simulink model "sim_validation_6DoF_3DoF"  (R2025a)
settings: Solver=VariableStepAuto  StartTime=0.0  StopTime=tf  RelTol=1e-12  AbsTol=1e-12
values from neighbouring files (symbols this model uses):
  alpha = 0.5086    [3DoF_deterministic_Workspace.mat]    (also in Compressed_Time_Step_2dof_Experiment.mat; Copy_of_Deterministic_6DoF.m; Copy_of_Deterministic_6DoF_quat.m; Copy_of_SCP_Earth_Mars_transfer_GA_uniform_adaptive.m = 1)
  I = 0.15    [3DoF_deterministic_Workspace.mat]    (also in Copy_of_DQG_6DoF_fixedtf.m = [4.2; 4.2; 0.6]; Copy_of_Deterministic_6DoF.m = [50000; 150000; 150000] * (1e-3) ^ 2; Copy_of_Deterministic_6DoF_quat.m = [50000; 150000; 150000] * (1e-3) ^ 2; DQG_6DoF.m = [4.2; 4.2; 0.6])
  I_matrix = diag([I/5, I, I])    [Deterministic_3DoF_with_mass_convexified_reynolds.m]    (also in Deterministic_3DoF_with_mass_convexified_takeoffdivert.m; Deterministic_6DoF.m = diag(I); Deterministic_6DoF_reynolds.m = diag(I); Deterministic_6DoF_reynolds_quat_alphabeta.m = diag(I))
  input_vector = 1:nu    [Deterministic_3DoF_with_mass_convexified_reynolds.m]    (also in Deterministic_3DoF_with_mass_convexified_takeoffdivert.m; Deterministic_3DoF_with_mass_polar.m; Deterministic_6DoF.m; Deterministic_6DoF_reynolds.m)
  L = 0.003    [3DoF_deterministic_Workspace.mat]    (also in Compressed_Time_Step_2dof_Experiment.mat; Copy_of_DQG_6DoF_fixedtf.m = 1; Copy_of_Deterministic_6DoF.m; Copy_of_Deterministic_6DoF_quat.m)
  m_0 = 2100    [3DoF_deterministic_Workspace.mat]    (also in Compressed_Time_Step_2dof_Experiment.mat = 2000; Copy_of_Deterministic_6DoF.m = 2600; Copy_of_Deterministic_6DoF_quat.m = 2600; Copy_of_SCP_Earth_Mars_transfer_GA_uniform_adaptive.m = 1)
  m_dry = 1500    [3DoF_deterministic_Workspace.mat]    (also in Copy_of_Deterministic_6DoF.m = 2000; Copy_of_Deterministic_6DoF_quat.m = 2000; Deterministic_3DoF.m = 2000; Deterministic_3DoF_with_mass.m)
  m_wet = 600    [3DoF_deterministic_Workspace.mat]    (also in Copy_of_Deterministic_6DoF.m; Copy_of_Deterministic_6DoF_quat.m; Deterministic_3DoF.m; Deterministic_3DoF_with_mass.m)
  r_0_6DoF = [r_0(1); 0; r_0(2)]    [Deterministic_3DoF_with_mass_convexified_reynolds.m]    (also in Deterministic_3DoF_with_mass_convexified_takeoffdivert.m; Deterministic_6DoF.m = r_0; Deterministic_6DoF_reynolds.m = r_0; Deterministic_6DoF_reynolds_quat_alphabeta.m = r_0)
  rpy_0_6DoF = [0; theta_0; 0]    [Deterministic_3DoF_with_mass_convexified_reynolds.m]    (also in Deterministic_3DoF_with_mass_convexified_takeoffdivert.m; Deterministic_6DoF.m = dcm2angle(angle2dcm(theta1_0, theta2_0, theta3_0,"XYX"), "ZY; Deterministic_6DoF_reynolds.m = dcm2angle(angle2dcm(theta1_0, theta2_0, theta3_0,"XYX"), "ZY; Deterministic_6DoF_reynolds_quat_alphabeta.m = [theta_3; theta_1; theta_2])
  v_0_b_6DoF = [v_0_b(1); 0; v_0_b(2)]    [Deterministic_3DoF_with_mass_convexified_reynolds.m]    (also in Deterministic_3DoF_with_mass_convexified_takeoffdivert.m; Deterministic_6DoF.m = v_0_b; Deterministic_6DoF_reynolds.m = v_0_b; Deterministic_6DoF_reynolds_quat_alphabeta.m = quat_rot(q_conj(q_0), v_0))
  w_0_6DoF = [0; w_0; 0]    [Deterministic_3DoF_with_mass_convexified_reynolds.m]    (also in Deterministic_3DoF_with_mass_convexified_takeoffdivert.m; Deterministic_6DoF.m = w_0; Deterministic_6DoF_reynolds.m = w_0; Deterministic_6DoF_reynolds_quat_alphabeta.m = w_0)
  x_0_6DoF = [r_0_6DoF; v_0_6DoF; rpy_0_6DoF; w_0_6DoF; log(m_0)]    [Deterministic_3DoF_with_mass_convexified_reynolds.m]    (also in Deterministic_3DoF_with_mass_convexified_takeoffdivert.m; Deterministic_6DoF.m = [r_0_6DoF; v_0_6DoF; rpy_0_6DoF; w_0_6DoF]; Deterministic_6DoF_reynolds.m = [r_0_6DoF; v_0_6DoF; rpy_0_6DoF; w_0_6DoF]; Deterministic_6DoF_reynolds_quat_alphabeta.m = x_0)
undefined symbols (not defined in the file or in its folder): construct_dual_quat
libraries: sharedtransform x2, simulink_extras x2, aerolibanim x1, aerolibobsolete x1, aerolibanimutils x1
settings Model: Creator=thatf  LastModifiedBy=thatf

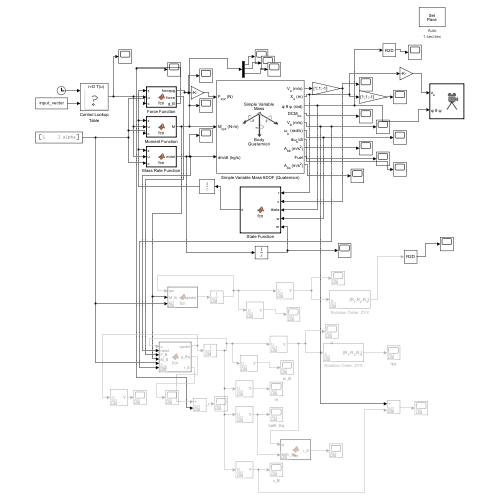
[thumbnail: Simulink's stored preview of the top-level diagram]
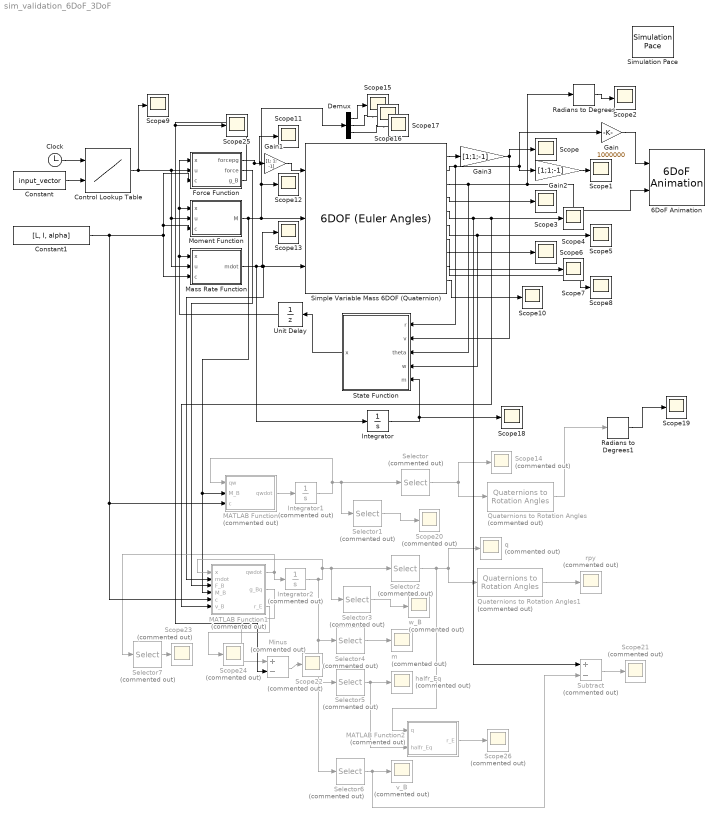
== system sim_validation_6DoF_3DoF ==
  6DoF Animation : aerolibanim/6DoF Animation  u1=[-1000 1000 -1000 1000 -5000 50]  u2=0.05  u3=100  u4=[0 0 0]  u5=Fly alongside  u6=[0 1000 0]  u7=80  u8=on
  Clock : Clock
  Constant : Constant  Value=input_vector
  Constant1 : Constant  Value=[L, I, alpha]
  Control Lookup Table : Lookup_n-D  BreakpointsForDimension1=opt_time'  BreakpointsForDimension2=input_vector  Table=control_inputs'  InternalRulePriority=Speed  RndMeth=Simplest
      settings: InputPortMap=u0,u1
  Demux : Demux  Outputs=3
  Force Function : MATLAB Function  TreatAsAtomicUnit=on
  Gain : Gain  Gain=1000000
  Gain1 : Gain  Gain=[1; 1; -1]
  Gain2 : Gain  Gain=[1;1;-1]
  Gain3 : Gain  Gain=[1;1;-1]
  Integrator : Integrator  InitialCondition=m_0
  Integrator1 : Integrator  Commented=on  InitialCondition=[[0 1 0 0; 0 0 1 0; 0 0 0 1; 1 0 0 0] * angle2quat(rpy_0_6DoF(1), rpy_0_6DoF(2), rpy_0_6DoF(3))'; w_0_6DoF]
  Integrator2 : Integrator  Commented=on  InitialCondition=[m_0; construct_dual_quat([0 1 0 0; 0 0 1 0; 0 0 0 1; 1 0 0 0] * angle2quat(rpy_0_6DoF(1), rpy_0_6DoF(2), rpy_0_6DoF(3))', r_0_6DoF); w_0_6DoF; v_0_b_6DoF]
  MATLAB Function : MATLAB Function  Commented=on  TreatAsAtomicUnit=on
  MATLAB Function1 : MATLAB Function  Commented=on  TreatAsAtomicUnit=on
  MATLAB Function2 : MATLAB Function  Commented=on  TreatAsAtomicUnit=on
  Mass Rate Function : MATLAB Function  TreatAsAtomicUnit=on
  Minus : Sum  Commented=on  Inputs=+-
  Moment Function : MATLAB Function  TreatAsAtomicUnit=on
  Quaternions to Rotation Angles : sharedtransform/Quaternions to Rotation Angles  Commented=on  rotationOrder=ZYX  aMode=aMode
  Quaternions to Rotation Angles1 : sharedtransform/Quaternions to Rotation Angles  Commented=on  rotationOrder=ZYX  aMode=aMode
  Radians to Degrees : simulink_extras/Transformations/Radians to Degrees
  Radians to Degrees1 : simulink_extras/Transformations/Radians to Degrees
  Scope{,1..13,15..19,25} (20 alike) : Scope
      Scope settings: ActiveDisplayYMinimum=-0.67191  ActiveDisplayYMaximum=-0.0103
      Scope1 settings: ActiveDisplayYMinimum=-7.33016  ActiveDisplayYMaximum=5.92557
      Scope10 settings: ActiveDisplayYMinimum=-0.01134  ActiveDisplayYMaximum=0.0087  DataLoggingVariableName=ScopeData2
      Scope11 settings: ActiveDisplayYMinimum=-25.88331  ActiveDisplayYMaximum=91.30016
      Scope12 settings: ActiveDisplayYMinimum=-0.01345  ActiveDisplayYMaximum=0.01341  DataLoggingVariableName=ScopeData2
      Scope13 settings: ActiveDisplayYMinimum=-33.22212  ActiveDisplayYMaximum=-15.43213  DataLoggingVariableName=ScopeData3
      Scope15 settings: ActiveDisplayYMinimum=-1  ActiveDisplayYMaximum=1  DataLoggingVariableName=ScopeData2
      Scope16 settings: ActiveDisplayYMinimum=-0.01345  ActiveDisplayYMaximum=0.01341  DataLoggingVariableName=ScopeData3
      Scope17 settings: ActiveDisplayYMinimum=-1  ActiveDisplayYMaximum=1  DataLoggingVariableName=ScopeData4
      Scope18 settings: ActiveDisplayYMinimum=1344.12679  ActiveDisplayYMaximum=2183.98591  DataLoggingVariableName=ScopeData5
      Scope19 settings: ActiveDisplayYMinimum=-1  ActiveDisplayYMaximum=1  DataLoggingVariableName=ScopeData2
      Scope2 settings: ActiveDisplayYMinimum=-225  ActiveDisplayYMaximum=225  DataLoggingVariableName=ScopeData2
      Scope25 settings: ActiveDisplayYMinimum=-0.01099  ActiveDisplayYMaximum=0.01074  DataLoggingVariableName=ScopeData15
      Scope3 settings: ActiveDisplayYMinimum=-1.25  ActiveDisplayYMaximum=1.25  DataLoggingVariableName=ScopeData3
      Scope4 settings: ActiveDisplayYMinimum=-0.68624  ActiveDisplayYMaximum=0.36359  DataLoggingVariableName=ScopeData4
      Scope5 settings: ActiveDisplayYMinimum=-0.26753  ActiveDisplayYMaximum=0.38262  DataLoggingVariableName=ScopeData5
      Scope6 settings: ActiveDisplayYMinimum=-0.08967  ActiveDisplayYMaximum=0.08939  DataLoggingVariableName=ScopeData6
      Scope7 settings: ActiveDisplayYMinimum=-0.18108  ActiveDisplayYMaximum=0.11428  DataLoggingVariableName=ScopeData7
      Scope8 settings: ActiveDisplayYMinimum=-0.125  ActiveDisplayYMaximum=1.125  DataLoggingVariableName=ScopeData8
      Scope9 settings: ActiveDisplayYMinimum=-0.00667  ActiveDisplayYMaximum=0.03493
  Scope{14,20..24,26} (7 alike) : Scope  Commented=on
      Scope14 settings: ActiveDisplayYMinimum=-0.12098  ActiveDisplayYMaximum=1.08883
      Scope20 settings: ActiveDisplayYMinimum=-0.38229  ActiveDisplayYMaximum=0.26726  DataLoggingVariableName=ScopeData3
      Scope21 settings: ActiveDisplayYMinimum=-0.04069  ActiveDisplayYMaximum=0.03672  DataLoggingVariableName=ScopeData11
      Scope22 settings: ActiveDisplayYMinimum=-6E-5  ActiveDisplayYMaximum=9E-5  DataLoggingVariableName=ScopeData12
      Scope23 settings: ActiveDisplayYMinimum=-0.03752  ActiveDisplayYMaximum=0.04457  DataLoggingVariableName=ScopeData13
      Scope24 settings: ActiveDisplayYMinimum=-0.64016  ActiveDisplayYMaximum=5.18224  DataLoggingVariableName=ScopeData14
      Scope26 settings: ActiveDisplayYMinimum=-5.29494  ActiveDisplayYMaximum=1.65449  DataLoggingVariableName=ScopeData9
  Selector : Selector  Commented=on  InputPortWidth=7  IndexOptions=Index vector (dialog)  Indices=[4 1 2 3]  OutputSizes=1
  Selector1 : Selector  Commented=on  InputPortWidth=7  IndexOptions=Index vector (dialog)  Indices=[5:7]  OutputSizes=1
  Selector2 : Selector  Commented=on  InputPortWidth=15  IndexOptions=Index vector (dialog)  Indices=[5 2 3 4]  OutputSizes=1
  Selector3 : Selector  Commented=on  InputPortWidth=15  IndexOptions=Index vector (dialog)  Indices=[10:12]  OutputSizes=1
  Selector4 : Selector  Commented=on  InputPortWidth=15  IndexOptions=Index vector (dialog)  Indices=[1]  OutputSizes=1
  Selector5 : Selector  Commented=on  InputPortWidth=15  IndexOptions=Index vector (dialog)  Indices=[6:9]  OutputSizes=1
  Selector6 : Selector  Commented=on  InputPortWidth=15  IndexOptions=Index vector (dialog)  Indices=[13:15]  OutputSizes=1
  Selector7 : Selector  Commented=on  InputPortWidth=15  IndexOptions=Index vector (dialog)  Indices=[13:15]  OutputSizes=1
  Simple Variable Mass 6DOF (Quaternion) : aerolibobsolete/6DOF (Euler Angles)  units=Metric (MKS)  mtype=Simple Variable  rep=Quaternion  xme_0=r_0_6DoF .* [1; 1; -1]  Vm_0=v_0_b_6DoF .* [1; 1; -1]  eul_0=rpy_0_6DoF  pm_0=w_0_6DoF  mass_0=m_0  mass_e=m_dry  mass_f=m_wet + m_dry  inertia=eye(3)  inertia_e=I_matrix - 1e-12  inertia_f=I_matrix  k_quat=1.0  vre_flag=off  abi_flag=on  aMode=0  xme_statename=''  Vm_statename=''  eul_statename=''  quat_statename=''  pm_statename=''  mass_statename=''
  Simulation Pace : aerolibanimutils/Simulation Pace  SimulationPace=1  SleepMode=Auto  OutputPaceError=off  SampleTime=1/30
  State Function : MATLAB Function  TreatAsAtomicUnit=on
  Subtract : Sum  Commented=on  Inputs=+-
  Unit Delay : UnitDelay  InitialCondition=x_0_6DoF  SampleTime=-1  HasFrameUpgradeWarning=on
  halfr_Eq : Scope  Commented=on
      settings: ActiveDisplayYMinimum=-2.39  ActiveDisplayYMaximum=1.59146  DataLoggingVariableName=ScopeData8
  m : Scope  Commented=on
      settings: ActiveDisplayYMinimum=1344.12679  ActiveDisplayYMaximum=2183.98591  DataLoggingVariableName=ScopeData7
  q : Scope  Commented=on
      settings: ActiveDisplayYMinimum=-0.12098  ActiveDisplayYMaximum=1.08883  DataLoggingVariableName=ScopeData4
  rpy : Scope  Commented=on
      settings: ActiveDisplayYMinimum=-0.3927  ActiveDisplayYMaximum=3.53429  DataLoggingVariableName=ScopeData6
  v_B : Scope  Commented=on
      settings: ActiveDisplayYMinimum=-0.34837  ActiveDisplayYMaximum=0.07536  DataLoggingVariableName=ScopeData10
  w_B : Scope  Commented=on
      settings: ActiveDisplayYMinimum=-0.38229  ActiveDisplayYMaximum=0.26726  DataLoggingVariableName=ScopeData5
  wires:
  Mass Rate Function/1(mdot) -> MATLAB Function1/2(mdot), Simple Variable Mass 6DOF (Quaternion)/3, Scope13/1, Integrator/1
  Simple Variable Mass 6DOF (Quaternion)/3 -> State Function/3(theta), 6DoF Animation/2, Radians to Degrees/1
  Simple Variable Mass 6DOF (Quaternion)/4 -> Scope3/1
  Simple Variable Mass 6DOF (Quaternion)/6 -> State Function/4(w), Scope5/1
  Simple Variable Mass 6DOF (Quaternion)/7 -> Scope6/1
  Simple Variable Mass 6DOF (Quaternion)/8 -> Scope7/1
  Simple Variable Mass 6DOF (Quaternion)/9 -> Scope8/1
  Simple Variable Mass 6DOF (Quaternion)/2 -> Gain2/1, Gain/1, State Function/1(r)
  Constant/1 -> Control Lookup Table/2
  Clock/1 -> Control Lookup Table/1
  Control Lookup Table/1 -> Scope9/1, Force Function/2(u), Mass Rate Function/2(u), Moment Function/2(u)
  Integrator/1 -> State Function/5(m), Scope18/1
  Simple Variable Mass 6DOF (Quaternion)/10 -> Scope10/1
  Gain/1 -> 6DoF Animation/1
  State Function/1(x) -> Unit Delay/1
  Demux/2 -> Scope16/1
  Demux/1 -> Scope15/1
  Demux/3 -> Scope17/1
  Radians to Degrees/1 -> Scope2/1
  Gain1/1 -> Simple Variable Mass 6DOF (Quaternion)/1
  Gain2/1 -> Scope1/1
  Simple Variable Mass 6DOF (Quaternion)/1 -> Gain3/1
  Gain3/1 -> State Function/2(v), Scope/1
  Unit Delay/1 -> Force Function/1(x), Moment Function/1(x), Mass Rate Function/1(x)
  Integrator1/1 -> Selector1/1, Selector/1, MATLAB Function/1(qw)
  MATLAB Function/1(qwdot) -> Integrator1/1
  Selector/1 -> Quaternions to Rotation Angles/1, Scope14/1
  Quaternions to Rotation Angles/1 -> Radians to Degrees1/1
  Radians to Degrees1/1 -> Scope19/1
  Selector1/1 -> Scope20/1
  MATLAB Function1/1(qwdot) -> Integrator2/1, Selector7/1
  Selector3/1 -> w_B/1
  Selector2/1 -> MATLAB Function2/1(q), Quaternions to Rotation Angles1/1, q/1
  Moment Function/1(M) -> MATLAB Function1/4(M_B), MATLAB Function/2(M_B), Demux/1, Scope12/1, Simple Variable Mass 6DOF (Quaternion)/2
  Constant1/1 -> MATLAB Function1/5(c), MATLAB Function/3(c), Moment Function/3(c), Force Function/3(c), Mass Rate Function/3(c)
  Integrator2/1 -> Selector6/1, Selector5/1, Selector4/1, Selector3/1, Selector2/1, MATLAB Function1/1(x)
  Quaternions to Rotation Angles1/1 -> rpy/1
  Selector4/1 -> m/1
  Selector5/1 -> MATLAB Function2/2(halfr_Eq), halfr_Eq/1
  MATLAB Function2/1(r_E) -> Scope26/1
  Selector6/1 -> Subtract/2, v_B/1
  Subtract/1 -> Scope21/1
  Simple Variable Mass 6DOF (Quaternion)/5 -> MATLAB Function1/6(v_B), Scope4/1, Subtract/1
  Force Function/1(forcepg) -> Scope11/1, Gain1/1
  Force Function/2(force) -> MATLAB Function1/3(F_B)
  MATLAB Function1/2(g_Bq) -> Minus/1
  Force Function/3(g_B) -> Scope25/1, Minus/2
  Minus/1 -> Scope22/1
  Selector7/1 -> Scope23/1
  MATLAB Function1/3(r_E) -> Scope24/1

== matlab function sim_validation_6DoF_3DoF/Moment Function ==
  data: x input; u input; M output; c input
function M = fcn(x, u, c)

m = exp(x(end));
a = u(1:2);
L = c(1);

T = m * a;

M = [0, 0, 0; 0, 0, 1; 0, 0, 0] * cross([-L; 0; 0], [T; 0]);

== matlab function sim_validation_6DoF_3DoF/Force Function ==
  data: forcepg output; x input; u input; force output; c input; g_B output
function [forcepg,force, g_B] = fcn(x, u, c)
rpy = x(7:9);
m = exp(x(end));
a = u(1:2);

R = angle2dcm(rpy(1), rpy(2), rpy(3), "ZYX");
g = 9.81e-3;

g_B = R' * [0; 0; g]

forcepg = [1, 0; 0, 0; 0, 1] * m * a - R' * [0; 0; g] * m;

force = [1, 0; 0, 0; 0, 1] * m * a;

== matlab function sim_validation_6DoF_3DoF/Mass Rate Function ==
  data: x input; u input; mdot output; c input
function mdot = fcn(x, u, c)

m = exp(x(end));
a = norm(u(1:2));

T = a * m;

alpha = c(3);

mdot = -alpha * T;

== matlab function sim_validation_6DoF_3DoF/State Function ==
  data: r input; x output; v input; theta input; w input; m input
function x = fcn(r, v, theta, w, m)

x = [r; v; theta; w; log(m)];

== matlab function sim_validation_6DoF_3DoF/MATLAB Function ==
  data: qw input; qwdot output; M_B input; c input
function qwdot = fcn(qw, M_B, c)

q = qw(1:4);
w_B = qw(5:7);

I = c(2);
J = diag([I; I; I]);

qdot = 1/2 * q_mul(q, [w_B; 0]);

wdot = inv(J) * (M_B - skew(w_B) * J * w_B);

qwdot = [qdot; wdot];

== matlab function sim_validation_6DoF_3DoF/MATLAB Function1 ==
  data: x input; mdot input; F_B input; qwdot output; M_B input; c input; g_Bq output; v_B input; r_E output
function [qwdot,g_Bq,r_E] = fcn(x, mdot, F_B, M_B, c, v_B)

m = x(1);
q = x(2:5);
qq = x(2:9);
w_B = x(10:12);
v_B = x(13:15);
w = x(10:15);

v_B = quat_rot(q, quat_rot(q_conj(q), v_B) .* [1; 1; -1]);

r_E = q_mul((x(6:9) * 2), q_conj(q));

I = c(2);
I_matrix = diag([I; I; I]);

qqdot = 1/2 * qq_mul(qq, [w_B; 0; v_B; 0]);

J = [zeros(3, 3), m * eye(3); I_matrix, zeros(3, 3)];

g_Bq = quat_rot(q, [0; 0; 9.81e-3]) .* [-1; 1; 1]

wdot = inv(J) * ([F_B; M_B] - qq_cross_matrix(w) * J * w + [m * quat_rot(q, [0; 0; 9.81e-3]) .* [1; 1; 1]; [0; 0; 0]]);

qwdot = [mdot; qqdot; wdot];
end
function qq_cross = qq_cross_matrix(qq)
    qq_cross = [skew(qq(1:3)), zeros(3, 3); skew(qq(4:6)), skew(qq(1:3))];
end

== matlab function sim_validation_6DoF_3DoF/MATLAB Function2 ==
  data: q input; halfr_Eq input; r_E output
function r_E = fcn(q, halfr_Eq)

r_E = 2 * q_mul([halfr_Eq; 0], q_conj(q));
